simulink model "xeng_8ant"  (Simulink 7.9)
settings: Solver=ode45  StartTime=0.0  StopTime=10.0  RelTol=1e-3
undefined symbols (not defined in the file): casper_library_multipliers, cmult_4bit_em
libraries: xbsIndex_r4 x761, xbsReplacements_r4 x72, casper_library_misc x19, casper_library_correlator x2, casper_library_delays x1
(part 1 of 9)
settings Model: Creator=tfiliba  LastModifiedBy=tfiliba

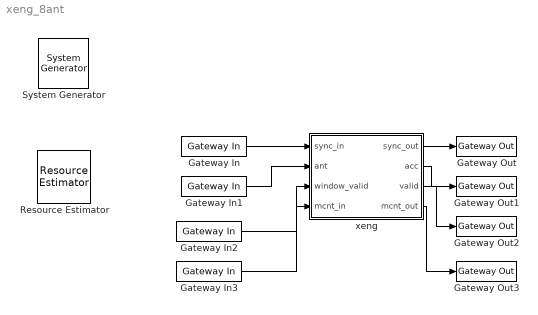
== system xeng_8ant ==
  " System Generator" : xbsIndex_r4/ System Generator  Tag=genX  xilinxfamily=virtex5  part=xc5vsx95t  speed=-1  package=ff1136  synthesis_tool=XST  clock_wrapper=Clock Enables  directory=./netlist  proj_type=Project Navigator  Synth_file=XST Defaults  Impl_file=ISE Defaults  testbench=off  simulink_period=1  sysclk_period=10  dcm_input_clock_period=10  incr_netlist=off  trim_vbits=Everywhere in SubSystem  dbl_ovrd=According to Block Masks  core_generation=According to Block Masks  run_coregen=off  deprecated_control=off  eval_field=0  block_type=sysgen
  Gateway In : xbsIndex_r4/Gateway In  gui_display_data_type=Boolean  arith_type=Boolean  n_bits=16  bin_pt=14  preci_type=Single  exp_width=8  frac_width=24  quantization="Round  (unbiased: +/- Inf)"  overflow=Saturate  period=1  dbl_ovrd=off  timing_constraint=None  locs_specified=off  LOCs={}  UseAsADC=off  ADCChannel='1'  inherit_from_input=off  hdl_port=on  block_type=gatewayin
      settings: xl_area=[0 0 0 0 1 0 0]
  Gateway In1 : xbsIndex_r4/Gateway In  gui_display_data_type=Fixed-point  arith_type="Signed  (2's comp)"  n_bits=32  bin_pt=0  preci_type=Single  exp_width=8  frac_width=24  quantization="Round  (unbiased: +/- Inf)"  overflow=Saturate  period=1  dbl_ovrd=off  timing_constraint=None  locs_specified=off  LOCs={}  UseAsADC=off  ADCChannel='1'  inherit_from_input=off  hdl_port=on  block_type=gatewayin
      settings: xl_area=[0 0 0 0 32 0 0]
  Gateway In2 : xbsIndex_r4/Gateway In  gui_display_data_type=Boolean  arith_type=Boolean  n_bits=4  bin_pt=3  preci_type=Single  exp_width=8  frac_width=24  quantization="Round  (unbiased: +/- Inf)"  overflow=Saturate  period=1  dbl_ovrd=off  timing_constraint=None  locs_specified=off  LOCs={}  UseAsADC=off  ADCChannel='1'  inherit_from_input=off  hdl_port=on  block_type=gatewayin
      settings: xl_area=[0 0 0 0 1 0 0]
  Gateway In3 : xbsIndex_r4/Gateway In  gui_display_data_type=Boolean  arith_type=Boolean  n_bits=4  bin_pt=3  preci_type=Single  exp_width=8  frac_width=24  quantization="Round  (unbiased: +/- Inf)"  overflow=Saturate  period=1  dbl_ovrd=off  timing_constraint=None  locs_specified=off  LOCs={}  UseAsADC=off  ADCChannel='1'  inherit_from_input=off  hdl_port=on  block_type=gatewayin
      settings: xl_area=[0 0 0 0 1 0 0]
  Gateway Out{,1..3} (4 alike) : xbsIndex_r4/Gateway Out  inherit_from_input=off  hdl_port=on  timing_constraint=None  locs_specified=off  LOCs={}  UseAsDAC=off  DACChannel='1'  block_type=gatewayout
      Gateway Out settings: xl_area=[0 0 0 0 1 0 0]
      Gateway Out1 settings: xl_area=[0 0 0 0 16 0 0]
      Gateway Out2 settings: xl_area=[0 0 0 0 1 0 0]
      Gateway Out3 settings: xl_area=[0 0 0 0 1 0 0]
  Resource Estimator : xbsIndex_r4/Resource Estimator  Tag=resEstTag  Slices=4251  FFs=5942  BRAMs=24  LUTs=5653  IOBs=39  EBMs=144  TBUFs=0  xl_use_estimator_area=off  est_options=Estimate  xl_estimator_area="[ 4251  5942    24  5653    39   144     0 ]"  block_type=resource_estimator
      settings: AttributesFormatString=Resource\nEstimator
  xeng : Subsystem  AncestorBlock=casper_library_correlator/xeng  mask(xeng){n_ants=8, n_bits=4, acc_len=128, demux_factor=8, add_latency=1, mult_latency=1, bram_latency=2, use_ded_mult=1, use_bram_delay=1}
      mask prompts: n_ants "Number of antennas"; n_bits "Bit-width of samples in"; acc_len "Accumulation length"; add_latency "Adder latency"; mult_latency "Multiplier latency"; bram_latency "BRAM latency"; use_ded_mult "Implementation: Multiplier type (0=slices 1=embedded 2=bram)"; use_bram_delay "Implementation: Delay type (0=SLR, 1=BRAM)"
      mask help: CASPER X engine with added internal valid data masking functionality, descramble and integral demux. Based on Aaron Parsons' and Lynn Urry's original X engine design.
      mask init:
      | xeng_init(gcb, ...
      |     'n_ants', n_ants, ...
      |     'n_bits', n_bits, ...
      |     'acc_len', acc_len, ...
      |     'demux_factor', demux_factor, ...
      |     'add_latency', add_latency, ...
      |     'mult_latency', mult_latency, ...
      |     'bram_latency', bram_latency, ...
      |     'use_ded_mult', use_ded_mult, ...
      |     'use_bram_delay', use_bram_delay);
      settings: AttributesFormatString=n_ant=8, bits=4, mult=1, bram=1
      mask StyleString: edit,edit,edit,popup(1|2|4|8),edit,edit,edit,edit,edit
  wires:
  Gateway In/1 -> xeng/1(sync_in)
  Gateway In1/1 -> xeng/2(ant)
  Gateway In2/1 -> xeng/3(window_valid)
  Gateway In3/1 -> xeng/4(mcnt_in)
  xeng/1(sync_out) -> Gateway Out/1
  xeng/2(acc) -> Gateway Out1/1
  xeng/3(valid) -> Gateway Out2/1
  xeng/4(mcnt_out) -> Gateway Out3/1

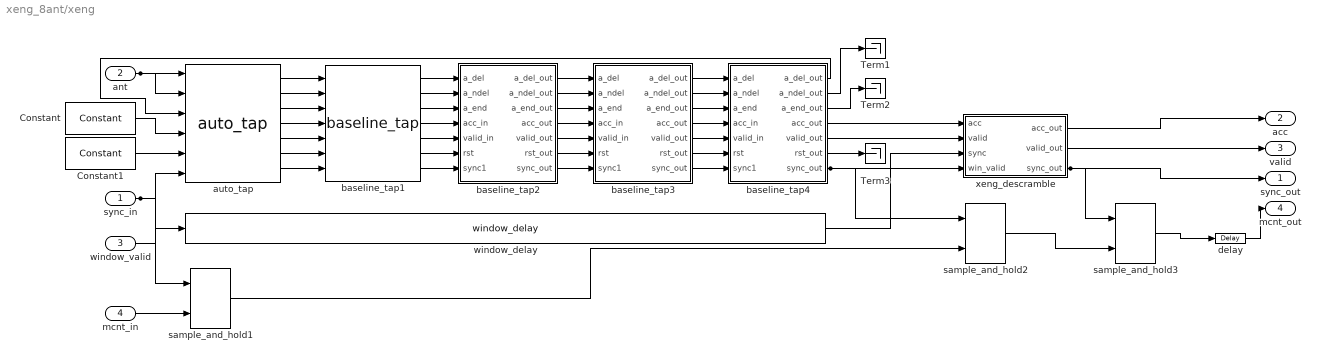
== system xeng_8ant/xeng ==
  sync_in : Inport
  ant : Inport  Port=2
  window_valid : Inport  Port=3
  mcnt_in : Inport  Port=4
  Constant : xbsIndex_r4/Constant  const=0  gui_display_data_type=Fixed-point  arith_type=Unsigned  n_bits=128  bin_pt=14  preci_type=Single  exp_width=8  frac_width=24  explicit_period=off  period=1  equ=P=C  opselect=C  inp2=PCIN>>17  opr=+  inp1=P  carry=CIN  dbl_ovrd=off  block_type=constant
  Constant1 : xbsIndex_r4/Constant  const=0  gui_display_data_type=Fixed-point  arith_type=Boolean  n_bits=1  bin_pt=14  preci_type=Single  exp_width=8  frac_width=24  explicit_period=off  period=1  equ=P=C  opselect=C  inp2=PCIN>>17  opr=+  inp1=P  carry=CIN  dbl_ovrd=off  block_type=constant
  Term1 : Terminator
  Term2 : Terminator
  Term3 : Terminator
  auto_tap : casper_library_correlator/auto_tap  n_ants=8  n_bits=4  acc_len=128  add_latency=1  mult_latency=1  bram_latency=2  use_ded_mult=1  use_bram_delay=1
      link override delay/Counter: use_behavioral_HDL=off  implementation=Fabric  use_rpm=off
      link override dual_pol_cmac/cmac1/cmult*/Resource Estimator: xl_estimator_area=[26 0 0 50 0 4 0]
      link override dual_pol_cmac/cmac2/cmult*/Resource Estimator: xl_estimator_area=[26 0 0 50 0 4 0]
      link override dual_pol_cmac/cmac3/cmult*/Resource Estimator: xl_estimator_area=[26 0 0 50 0 4 0]
      link override dual_pol_cmac/cmac4/cmult*/Resource Estimator: xl_estimator_area=[26 0 0 50 0 4 0]
      settings: AttributesFormatString=mult=1
      link override delay/Counter: xl_area=[8 10 0 13 0 0 0]
      link override delay/Single Port RAM: xl_area=[0 32 8 0 0 0 0]
      link override dual_pol_cmac/cmac1/Counter: xl_area=[6 7 0 9 0 0 0]
      link override dual_pol_cmac/cmac1/Delay: xl_area=[1 1 0 0 0 0 0]
      link override dual_pol_cmac/cmac1/Relational: xl_area=[2 1 0 4 0 0 0]
      link override dual_pol_cmac/cmac1/acc/Accumulator: xl_area=[8 16 0 16 0 0 0]
      link override dual_pol_cmac/cmac1/acc/Convert1: xl_area=[0 0 0 0 0 0 0]
      link override dual_pol_cmac/cmac1/acc/Convert2: xl_area=[0 0 0 0 0 0 0]
      link override dual_pol_cmac/cmac1/acc/Delay: xl_area=[0 0 0 0 0 0 0]
      link override dual_pol_cmac/cmac1/acc/Delay1: xl_area=[0 0 0 0 0 0 0]
      link override dual_pol_cmac/cmac1/acc/Mux2: xl_area=[16 32 0 16 0 0 0]
      link override dual_pol_cmac/cmac1/acc/Mux3: xl_area=[1 2 0 1 0 0 0]
      link override dual_pol_cmac/cmac1/acc1/Accumulator: xl_area=[8 16 0 16 0 0 0]
      link override dual_pol_cmac/cmac1/acc1/Convert1: xl_area=[0 0 0 0 0 0 0]
      link override dual_pol_cmac/cmac1/acc1/Convert2: xl_area=[0 0 0 0 0 0 0]
      link override dual_pol_cmac/cmac1/acc1/Delay: xl_area=[0 0 0 0 0 0 0]
      link override dual_pol_cmac/cmac1/acc1/Delay1: xl_area=[0 0 0 0 0 0 0]
      link override dual_pol_cmac/cmac1/acc1/Mux2: xl_area=[16 32 0 16 0 0 0]
      link override dual_pol_cmac/cmac1/acc1/Mux3: xl_area=[1 2 0 1 0 0 0]
      link override dual_pol_cmac/cmac1/cmult*/ac: xl_area=[4 0 0 8 0 1 0]
      link override dual_pol_cmac/cmac1/cmult*/ad: xl_area=[4 0 0 8 0 1 0]
      link override dual_pol_cmac/cmac1/cmult*/bc: xl_area=[4 0 0 8 0 1 0]
      link override dual_pol_cmac/cmac1/cmult*/bd: xl_area=[4 0 0 8 0 1 0]
      link override dual_pol_cmac/cmac1/cmult*/imag_sum: xl_area=[5 0 0 9 0 0 0]
      link override dual_pol_cmac/cmac1/cmult*/real_sum: xl_area=[5 0 0 9 0 0 0]
      link override dual_pol_cmac/cmac2/Counter: xl_area=[6 7 0 9 0 0 0]
      link override dual_pol_cmac/cmac2/Delay: xl_area=[1 1 0 0 0 0 0]
      link override dual_pol_cmac/cmac2/Relational: xl_area=[2 1 0 4 0 0 0]
      link override dual_pol_cmac/cmac2/acc/Accumulator: xl_area=[8 16 0 16 0 0 0]
      link override dual_pol_cmac/cmac2/acc/Convert1: xl_area=[0 0 0 0 0 0 0]
      link override dual_pol_cmac/cmac2/acc/Convert2: xl_area=[0 0 0 0 0 0 0]
      link override dual_pol_cmac/cmac2/acc/Delay: xl_area=[0 0 0 0 0 0 0]
      link override dual_pol_cmac/cmac2/acc/Delay1: xl_area=[0 0 0 0 0 0 0]
      link override dual_pol_cmac/cmac2/acc/Mux2: xl_area=[16 32 0 16 0 0 0]
      link override dual_pol_cmac/cmac2/acc/Mux3: xl_area=[1 2 0 1 0 0 0]
      link override dual_pol_cmac/cmac2/acc1/Accumulator: xl_area=[8 16 0 16 0 0 0]
      link override dual_pol_cmac/cmac2/acc1/Convert1: xl_area=[0 0 0 0 0 0 0]
      link override dual_pol_cmac/cmac2/acc1/Convert2: xl_area=[0 0 0 0 0 0 0]
      link override dual_pol_cmac/cmac2/acc1/Delay: xl_area=[0 0 0 0 0 0 0]
      link override dual_pol_cmac/cmac2/acc1/Delay1: xl_area=[0 0 0 0 0 0 0]
      link override dual_pol_cmac/cmac2/acc1/Mux2: xl_area=[16 32 0 16 0 0 0]
      link override dual_pol_cmac/cmac2/acc1/Mux3: xl_area=[1 2 0 1 0 0 0]
      link override dual_pol_cmac/cmac2/cmult*/ac: xl_area=[4 0 0 8 0 1 0]
      link override dual_pol_cmac/cmac2/cmult*/ad: xl_area=[4 0 0 8 0 1 0]
      link override dual_pol_cmac/cmac2/cmult*/bc: xl_area=[4 0 0 8 0 1 0]
      link override dual_pol_cmac/cmac2/cmult*/bd: xl_area=[4 0 0 8 0 1 0]
      link override dual_pol_cmac/cmac2/cmult*/imag_sum: xl_area=[5 0 0 9 0 0 0]
      link override dual_pol_cmac/cmac2/cmult*/real_sum: xl_area=[5 0 0 9 0 0 0]
      link override dual_pol_cmac/cmac3/Counter: xl_area=[6 7 0 9 0 0 0]
      link override dual_pol_cmac/cmac3/Delay: xl_area=[1 1 0 0 0 0 0]
      link override dual_pol_cmac/cmac3/Relational: xl_area=[2 1 0 4 0 0 0]
      link override dual_pol_cmac/cmac3/acc/Accumulator: xl_area=[8 16 0 16 0 0 0]
      link override dual_pol_cmac/cmac3/acc/Convert1: xl_area=[0 0 0 0 0 0 0]
      link override dual_pol_cmac/cmac3/acc/Convert2: xl_area=[0 0 0 0 0 0 0]
      link override dual_pol_cmac/cmac3/acc/Delay: xl_area=[0 0 0 0 0 0 0]
      link override dual_pol_cmac/cmac3/acc/Delay1: xl_area=[0 0 0 0 0 0 0]
      link override dual_pol_cmac/cmac3/acc/Mux2: xl_area=[16 32 0 16 0 0 0]
      link override dual_pol_cmac/cmac3/acc/Mux3: xl_area=[1 2 0 1 0 0 0]
      link override dual_pol_cmac/cmac3/acc1/Accumulator: xl_area=[8 16 0 16 0 0 0]
      link override dual_pol_cmac/cmac3/acc1/Convert1: xl_area=[0 0 0 0 0 0 0]
      link override dual_pol_cmac/cmac3/acc1/Convert2: xl_area=[0 0 0 0 0 0 0]
      link override dual_pol_cmac/cmac3/acc1/Delay: xl_area=[0 0 0 0 0 0 0]
      link override dual_pol_cmac/cmac3/acc1/Delay1: xl_area=[0 0 0 0 0 0 0]
      link override dual_pol_cmac/cmac3/acc1/Mux2: xl_area=[16 32 0 16 0 0 0]
      link override dual_pol_cmac/cmac3/acc1/Mux3: xl_area=[1 2 0 1 0 0 0]
      link override dual_pol_cmac/cmac3/cmult*/ac: xl_area=[4 0 0 8 0 1 0]
      link override dual_pol_cmac/cmac3/cmult*/ad: xl_area=[4 0 0 8 0 1 0]
      link override dual_pol_cmac/cmac3/cmult*/bc: xl_area=[4 0 0 8 0 1 0]
      link override dual_pol_cmac/cmac3/cmult*/bd: xl_area=[4 0 0 8 0 1 0]
      link override dual_pol_cmac/cmac3/cmult*/imag_sum: xl_area=[5 0 0 9 0 0 0]
      link override dual_pol_cmac/cmac3/cmult*/real_sum: xl_area=[5 0 0 9 0 0 0]
      link override dual_pol_cmac/cmac4/Counter: xl_area=[6 7 0 9 0 0 0]
      link override dual_pol_cmac/cmac4/Delay: xl_area=[1 1 0 0 0 0 0]
      link override dual_pol_cmac/cmac4/Relational: xl_area=[2 1 0 4 0 0 0]
      link override dual_pol_cmac/cmac4/acc/Accumulator: xl_area=[8 16 0 16 0 0 0]
      link override dual_pol_cmac/cmac4/acc/Convert1: xl_area=[0 0 0 0 0 0 0]
      link override dual_pol_cmac/cmac4/acc/Convert2: xl_area=[0 0 0 0 0 0 0]
      link override dual_pol_cmac/cmac4/acc/Delay: xl_area=[0 0 0 0 0 0 0]
      link override dual_pol_cmac/cmac4/acc/Delay1: xl_area=[0 0 0 0 0 0 0]
      link override dual_pol_cmac/cmac4/acc/Mux2: xl_area=[16 32 0 16 0 0 0]
      link override dual_pol_cmac/cmac4/acc/Mux3: xl_area=[1 2 0 1 0 0 0]
      link override dual_pol_cmac/cmac4/acc1/Accumulator: xl_area=[8 16 0 16 0 0 0]
      link override dual_pol_cmac/cmac4/acc1/Convert1: xl_area=[0 0 0 0 0 0 0]
      link override dual_pol_cmac/cmac4/acc1/Convert2: xl_area=[0 0 0 0 0 0 0]
      link override dual_pol_cmac/cmac4/acc1/Delay: xl_area=[0 0 0 0 0 0 0]
      link override dual_pol_cmac/cmac4/acc1/Delay1: xl_area=[0 0 0 0 0 0 0]
      link override dual_pol_cmac/cmac4/acc1/Mux2: xl_area=[16 32 0 16 0 0 0]
      link override dual_pol_cmac/cmac4/acc1/Mux3: xl_area=[1 2 0 1 0 0 0]
      link override dual_pol_cmac/cmac4/cmult*/ac: xl_area=[4 0 0 8 0 1 0]
      link override dual_pol_cmac/cmac4/cmult*/ad: xl_area=[4 0 0 8 0 1 0]
      link override dual_pol_cmac/cmac4/cmult*/bc: xl_area=[4 0 0 8 0 1 0]
      link override dual_pol_cmac/cmac4/cmult*/bd: xl_area=[4 0 0 8 0 1 0]
      link override dual_pol_cmac/cmac4/cmult*/imag_sum: xl_area=[5 0 0 9 0 0 0]
      link override dual_pol_cmac/cmac4/cmult*/real_sum: xl_area=[5 0 0 9 0 0 0]
      link override sync_delay/Counter: xl_area=[5 8 0 9 0 0 0]
      link override sync_delay/Logical: xl_area=[1 0 0 1 0 0 0]
      link override sync_delay/Mux: xl_area=[1 0 0 1 0 0 0]
      link override sync_delay/Relational: xl_area=[2 0 0 4 0 0 0]
      link override sync_delay/Relational1: xl_area=[2 0 0 4 0 0 0]
  baseline_tap1 : casper_library_correlator/baseline_tap  n_ants=8  ant_sep=1  n_bits=4  acc_len=128  add_latency=1  mult_latency=1  bram_latency=2  use_ded_mult=1  use_bram_delay=1
      link override delay/Counter: use_behavioral_HDL=off  implementation=Fabric  use_rpm=off
      link override dual_pol_cmac/cmac1/cmult*/Resource Estimator: xl_estimator_area=[26 0 0 50 0 4 0]
      link override dual_pol_cmac/cmac2/cmult*/Resource Estimator: xl_estimator_area=[26 0 0 50 0 4 0]
      link override dual_pol_cmac/cmac3/cmult*/Resource Estimator: xl_estimator_area=[26 0 0 50 0 4 0]
      link override dual_pol_cmac/cmac4/cmult*/Resource Estimator: xl_estimator_area=[26 0 0 50 0 4 0]
      settings: AttributesFormatString=ant_sep=1, mult=1, bram=1
      link override Convert: xl_area=[0 0 0 0 0 0 0]
      link override Counter: xl_area=[10 11 0 15 0 0 0]
      link override Delay1: xl_area=[1 1 0 0 0 0 0]
      link override Delay3: xl_area=[16 32 0 0 0 0 0]
      link override Delay7: xl_area=[16 32 0 0 0 0 0]
      link override Delay8: xl_area=[16 32 0 0 0 0 0]
      link override Mux: xl_area=[16 32 0 32 0 0 0]
      link override Relational: xl_area=[6 0 0 11 0 0 0]
      link override delay/Counter: xl_area=[6 7 0 9 0 0 0]
      link override delay/Single Port RAM: xl_area=[0 32 1 0 0 0 0]
      link override dual_pol_cmac/cmac1/Counter: xl_area=[6 7 0 9 0 0 0]
      link override dual_pol_cmac/cmac1/Delay: xl_area=[1 1 0 0 0 0 0]
      link override dual_pol_cmac/cmac1/Relational: xl_area=[2 1 0 4 0 0 0]
      link override dual_pol_cmac/cmac1/acc/Accumulator: xl_area=[8 16 0 16 0 0 0]
      link override dual_pol_cmac/cmac1/acc/Convert1: xl_area=[0 0 0 0 0 0 0]
      link override dual_pol_cmac/cmac1/acc/Convert2: xl_area=[0 0 0 0 0 0 0]
      link override dual_pol_cmac/cmac1/acc/Delay: xl_area=[0 0 0 0 0 0 0]
      link override dual_pol_cmac/cmac1/acc/Delay1: xl_area=[0 0 0 0 0 0 0]
      link override dual_pol_cmac/cmac1/acc/Mux2: xl_area=[16 32 0 16 0 0 0]
      link override dual_pol_cmac/cmac1/acc/Mux3: xl_area=[1 2 0 1 0 0 0]
      link override dual_pol_cmac/cmac1/acc1/Accumulator: xl_area=[8 16 0 16 0 0 0]
      link override dual_pol_cmac/cmac1/acc1/Convert1: xl_area=[0 0 0 0 0 0 0]
      link override dual_pol_cmac/cmac1/acc1/Convert2: xl_area=[0 0 0 0 0 0 0]
      link override dual_pol_cmac/cmac1/acc1/Delay: xl_area=[0 0 0 0 0 0 0]
      link override dual_pol_cmac/cmac1/acc1/Delay1: xl_area=[0 0 0 0 0 0 0]
      link override dual_pol_cmac/cmac1/acc1/Mux2: xl_area=[16 32 0 16 0 0 0]
      link override dual_pol_cmac/cmac1/acc1/Mux3: xl_area=[1 2 0 1 0 0 0]
      link override dual_pol_cmac/cmac1/cmult*/ac: xl_area=[4 0 0 8 0 1 0]
      link override dual_pol_cmac/cmac1/cmult*/ad: xl_area=[4 0 0 8 0 1 0]
      link override dual_pol_cmac/cmac1/cmult*/bc: xl_area=[4 0 0 8 0 1 0]
      link override dual_pol_cmac/cmac1/cmult*/bd: xl_area=[4 0 0 8 0 1 0]
      link override dual_pol_cmac/cmac1/cmult*/imag_sum: xl_area=[5 0 0 9 0 0 0]
      link override dual_pol_cmac/cmac1/cmult*/real_sum: xl_area=[5 0 0 9 0 0 0]
      link override dual_pol_cmac/cmac2/Counter: xl_area=[6 7 0 9 0 0 0]
      link override dual_pol_cmac/cmac2/Delay: xl_area=[1 1 0 0 0 0 0]
      link override dual_pol_cmac/cmac2/Relational: xl_area=[2 1 0 4 0 0 0]
      link override dual_pol_cmac/cmac2/acc/Accumulator: xl_area=[8 16 0 16 0 0 0]
      link override dual_pol_cmac/cmac2/acc/Convert1: xl_area=[0 0 0 0 0 0 0]
      link override dual_pol_cmac/cmac2/acc/Convert2: xl_area=[0 0 0 0 0 0 0]
      link override dual_pol_cmac/cmac2/acc/Delay: xl_area=[0 0 0 0 0 0 0]
      link override dual_pol_cmac/cmac2/acc/Delay1: xl_area=[0 0 0 0 0 0 0]
      link override dual_pol_cmac/cmac2/acc/Mux2: xl_area=[16 32 0 16 0 0 0]
      link override dual_pol_cmac/cmac2/acc/Mux3: xl_area=[1 2 0 1 0 0 0]
      link override dual_pol_cmac/cmac2/acc1/Accumulator: xl_area=[8 16 0 16 0 0 0]
      link override dual_pol_cmac/cmac2/acc1/Convert1: xl_area=[0 0 0 0 0 0 0]
      link override dual_pol_cmac/cmac2/acc1/Convert2: xl_area=[0 0 0 0 0 0 0]
      link override dual_pol_cmac/cmac2/acc1/Delay: xl_area=[0 0 0 0 0 0 0]
      link override dual_pol_cmac/cmac2/acc1/Delay1: xl_area=[0 0 0 0 0 0 0]
      link override dual_pol_cmac/cmac2/acc1/Mux2: xl_area=[16 32 0 16 0 0 0]
      link override dual_pol_cmac/cmac2/acc1/Mux3: xl_area=[1 2 0 1 0 0 0]
      link override dual_pol_cmac/cmac2/cmult*/ac: xl_area=[4 0 0 8 0 1 0]
      link override dual_pol_cmac/cmac2/cmult*/ad: xl_area=[4 0 0 8 0 1 0]
      link override dual_pol_cmac/cmac2/cmult*/bc: xl_area=[4 0 0 8 0 1 0]
      link override dual_pol_cmac/cmac2/cmult*/bd: xl_area=[4 0 0 8 0 1 0]
      link override dual_pol_cmac/cmac2/cmult*/imag_sum: xl_area=[5 0 0 9 0 0 0]
      link override dual_pol_cmac/cmac2/cmult*/real_sum: xl_area=[5 0 0 9 0 0 0]
      link override dual_pol_cmac/cmac3/Counter: xl_area=[6 7 0 9 0 0 0]
      link override dual_pol_cmac/cmac3/Delay: xl_area=[1 1 0 0 0 0 0]
      link override dual_pol_cmac/cmac3/Relational: xl_area=[2 1 0 4 0 0 0]
      link override dual_pol_cmac/cmac3/acc/Accumulator: xl_area=[8 16 0 16 0 0 0]
      link override dual_pol_cmac/cmac3/acc/Convert1: xl_area=[0 0 0 0 0 0 0]
      link override dual_pol_cmac/cmac3/acc/Convert2: xl_area=[0 0 0 0 0 0 0]
      link override dual_pol_cmac/cmac3/acc/Delay: xl_area=[0 0 0 0 0 0 0]
      link override dual_pol_cmac/cmac3/acc/Delay1: xl_area=[0 0 0 0 0 0 0]
      link override dual_pol_cmac/cmac3/acc/Mux2: xl_area=[16 32 0 16 0 0 0]
      link override dual_pol_cmac/cmac3/acc/Mux3: xl_area=[1 2 0 1 0 0 0]
      link override dual_pol_cmac/cmac3/acc1/Accumulator: xl_area=[8 16 0 16 0 0 0]
      link override dual_pol_cmac/cmac3/acc1/Convert1: xl_area=[0 0 0 0 0 0 0]
      link override dual_pol_cmac/cmac3/acc1/Convert2: xl_area=[0 0 0 0 0 0 0]
      link override dual_pol_cmac/cmac3/acc1/Delay: xl_area=[0 0 0 0 0 0 0]
      link override dual_pol_cmac/cmac3/acc1/Delay1: xl_area=[0 0 0 0 0 0 0]
      link override dual_pol_cmac/cmac3/acc1/Mux2: xl_area=[16 32 0 16 0 0 0]
      link override dual_pol_cmac/cmac3/acc1/Mux3: xl_area=[1 2 0 1 0 0 0]
      link override dual_pol_cmac/cmac3/cmult*/ac: xl_area=[4 0 0 8 0 1 0]
      link override dual_pol_cmac/cmac3/cmult*/ad: xl_area=[4 0 0 8 0 1 0]
      link override dual_pol_cmac/cmac3/cmult*/bc: xl_area=[4 0 0 8 0 1 0]
      link override dual_pol_cmac/cmac3/cmult*/bd: xl_area=[4 0 0 8 0 1 0]
      link override dual_pol_cmac/cmac3/cmult*/imag_sum: xl_area=[5 0 0 9 0 0 0]
      link override dual_pol_cmac/cmac3/cmult*/real_sum: xl_area=[5 0 0 9 0 0 0]
      link override dual_pol_cmac/cmac4/Counter: xl_area=[6 7 0 9 0 0 0]
      link override dual_pol_cmac/cmac4/Delay: xl_area=[1 1 0 0 0 0 0]
      link override dual_pol_cmac/cmac4/Relational: xl_area=[2 1 0 4 0 0 0]
      link override dual_pol_cmac/cmac4/acc/Accumulator: xl_area=[8 16 0 16 0 0 0]
      link override dual_pol_cmac/cmac4/acc/Convert1: xl_area=[0 0 0 0 0 0 0]
      link override dual_pol_cmac/cmac4/acc/Convert2: xl_area=[0 0 0 0 0 0 0]
      link override dual_pol_cmac/cmac4/acc/Delay: xl_area=[0 0 0 0 0 0 0]
      link override dual_pol_cmac/cmac4/acc/Delay1: xl_area=[0 0 0 0 0 0 0]
      link override dual_pol_cmac/cmac4/acc/Mux2: xl_area=[16 32 0 16 0 0 0]
      link override dual_pol_cmac/cmac4/acc/Mux3: xl_area=[1 2 0 1 0 0 0]
      link override dual_pol_cmac/cmac4/acc1/Accumulator: xl_area=[8 16 0 16 0 0 0]
      link override dual_pol_cmac/cmac4/acc1/Convert1: xl_area=[0 0 0 0 0 0 0]
      link override dual_pol_cmac/cmac4/acc1/Convert2: xl_area=[0 0 0 0 0 0 0]
      link override dual_pol_cmac/cmac4/acc1/Delay: xl_area=[0 0 0 0 0 0 0]
      link override dual_pol_cmac/cmac4/acc1/Delay1: xl_area=[0 0 0 0 0 0 0]
      link override dual_pol_cmac/cmac4/acc1/Mux2: xl_area=[16 32 0 16 0 0 0]
      link override dual_pol_cmac/cmac4/acc1/Mux3: xl_area=[1 2 0 1 0 0 0]
      link override dual_pol_cmac/cmac4/cmult*/ac: xl_area=[4 0 0 8 0 1 0]
      link override dual_pol_cmac/cmac4/cmult*/ad: xl_area=[4 0 0 8 0 1 0]
      link override dual_pol_cmac/cmac4/cmult*/bc: xl_area=[4 0 0 8 0 1 0]
      link override dual_pol_cmac/cmac4/cmult*/bd: xl_area=[4 0 0 8 0 1 0]
      link override dual_pol_cmac/cmac4/cmult*/imag_sum: xl_area=[5 0 0 9 0 0 0]
      link override dual_pol_cmac/cmac4/cmult*/real_sum: xl_area=[5 0 0 9 0 0 0]
  baseline_tap2 : Subsystem  AncestorBlock=casper_library_correlator/baseline_tap  mask(baseline_tap){n_ants=8, ant_sep=2, n_bits=4, acc_len=128, add_latency=1, mult_latency=1, bram_latency=2, use_ded_mult=1, use_bram_delay=1}
      mask prompts: n_ants "Number of antennas"; ant_sep "Antenna Seperation"; n_bits "number of input bits (per complex component)"; acc_len "accumulation length"; add_latency "Adder latency"; mult_latency "Multiplier latency"; bram_latency "BRAM latency"; use_ded_mult "Multiplier Type (0=slices 1=embedded 2=bram)"; use_bram_delay "Use BRAM delays"
      mask init:
      | fix_pnt_pos = (n_bits-1)*2;
      | bit_growth = ceil(log2(acc_len));
      | ant_bits = ceil(log2(n_ants));
      | n_bits_out = (2*n_bits + 1 + bit_growth);
      | 
      | baseline_tap_init(gcb, ...
      |     'ant_sep', ant_sep, ...
      |     'use_ded_mult', use_ded_mult, ...
      |     'use_bram_delay', use_bram_delay);
      settings: AttributesFormatString=ant_sep=2, mult=1, bram=1
  baseline_tap3 : Subsystem  AncestorBlock=casper_library_correlator/baseline_tap  mask(baseline_tap){n_ants=8, ant_sep=3, n_bits=4, acc_len=128, add_latency=1, mult_latency=1, bram_latency=2, use_ded_mult=1, use_bram_delay=1}
      mask prompts: n_ants "Number of antennas"; ant_sep "Antenna Seperation"; n_bits "number of input bits (per complex component)"; acc_len "accumulation length"; add_latency "Adder latency"; mult_latency "Multiplier latency"; bram_latency "BRAM latency"; use_ded_mult "Multiplier Type (0=slices 1=embedded 2=bram)"; use_bram_delay "Use BRAM delays"
      mask init: same as xeng_8ant/xeng/baseline_tap2
      settings: AttributesFormatString=ant_sep=3, mult=1, bram=1
  baseline_tap4 : Subsystem  AncestorBlock=casper_library_correlator/baseline_tap  mask(baseline_tap){n_ants=8, ant_sep=4, n_bits=4, acc_len=128, add_latency=1, mult_latency=1, bram_latency=2, use_ded_mult=1, use_bram_delay=1}
      mask prompts: n_ants "Number of antennas"; ant_sep "Antenna Seperation"; n_bits "number of input bits (per complex component)"; acc_len "accumulation length"; add_latency "Adder latency"; mult_latency "Multiplier latency"; bram_latency "BRAM latency"; use_ded_mult "Multiplier Type (0=slices 1=embedded 2=bram)"; use_bram_delay "Use BRAM delays"
      mask init: same as xeng_8ant/xeng/baseline_tap2
      settings: AttributesFormatString=ant_sep=4, mult=1, bram=1
  delay : xbsIndex_r4/Delay  rst=off  infoeditControl=Selection of Reset will increase slice count due to use of real FFs and instead of SRLs  en=off  latency=1  dbl_ovrd=off  reg_retiming=on  block_type=delay
  sample_and_hold1 : casper_library_misc/sample_and_hold  period=1024
      link override Counter4: xl_area=[7 11 0 11 0 0 0]
      link override Delay10: xl_area=[1 1 0 0 0 0 0]
      link override Logical: xl_area=[1 0 0 1 0 0 0]
      link override Register: xl_area=[1 1 0 0 0 0 0]
      link override Relational: xl_area=[6 0 0 12 0 0 0]
  sample_and_hold2 : casper_library_misc/sample_and_hold  period=1024
      link override Counter4: xl_area=[7 11 0 11 0 0 0]
      link override Delay10: xl_area=[1 1 0 0 0 0 0]
      link override Logical: xl_area=[1 0 0 1 0 0 0]
      link override Register: xl_area=[1 1 0 0 0 0 0]
      link override Relational: xl_area=[6 0 0 12 0 0 0]
  sample_and_hold3 : casper_library_misc/sample_and_hold  period=1024
      link override Counter4: xl_area=[7 11 0 11 0 0 0]
      link override Delay10: xl_area=[1 1 0 0 0 0 0]
      link override Logical: xl_area=[1 0 0 1 0 0 0]
      link override Register: xl_area=[1 1 0 0 0 0 0]
      link override Relational: xl_area=[6 0 0 12 0 0 0]
  window_delay : casper_library_delays/window_delay  delay=136
      link override Gateway Out2: xl_area=[0 0 0 0 1 0 0]
      link override Gateway Out3: xl_area=[0 0 0 0 1 0 0]
      link override Gateway Out55: xl_area=[0 0 0 0 1 0 0]
      link override Gateway Out56: xl_area=[0 0 0 0 1 0 0]
      link override Register: xl_area=[1 1 0 0 0 0 0]
      link override negedge/Delay: xl_area=[1 1 0 0 0 0 0]
      link override negedge/Inverter: xl_area=[0 0 0 0 0 0 0]
      link override negedge/Logical: xl_area=[1 0 0 1 0 0 0]
      link override posedge3/Delay: xl_area=[1 1 0 0 0 0 0]
      link override posedge3/Inverter: xl_area=[0 0 0 0 0 0 0]
      link override posedge3/Logical: xl_area=[1 0 0 1 0 0 0]
      link override sync_delay/Counter: xl_area=[5 8 0 9 0 0 0]
      link override sync_delay/Logical: xl_area=[1 0 0 1 0 0 0]
      link override sync_delay/Mux: xl_area=[1 0 0 1 0 0 0]
      link override sync_delay/Relational: xl_area=[2 0 0 4 0 0 0]
      link override sync_delay/Relational1: xl_area=[2 0 0 4 0 0 0]
      link override sync_delay1/Counter: xl_area=[5 8 0 9 0 0 0]
      link override sync_delay1/Logical: xl_area=[1 0 0 1 0 0 0]
      link override sync_delay1/Mux: xl_area=[1 0 0 1 0 0 0]
      link override sync_delay1/Relational: xl_area=[2 0 0 4 0 0 0]
      link override sync_delay1/Relational1: xl_area=[2 0 0 4 0 0 0]
  xeng_descramble : Subsystem  AncestorBlock=casper_library_correlator/xeng_descramble  mask(xeng_descramble){num_ants=8, n_bits=4, acc_len=128, demux_factor=8}
      mask prompts: num_ants "Number of Antennas"; n_bits "Input Bitwidth"; acc_len "X engine accumulation length"; demux_factor "Demux Factor"
      mask help:
      | NOT TESTED FOR non-2^N antennas.
      |
      | Descrambles X engine output. Optionally demuxes output.
      mask init:
      | num_taps = floor(num_ants/2) + 1;
      | ant_bits = ceil(log2(num_ants));
      | num_validins = num_ants*num_taps;
      | validin_bits = floor(log2(num_validins))+1;
      | demux_bits = floor(log2(demux_factor))+1;
      | acc_len_bits = floor(log2(acc_len))+1;
      | num_ants_bits = floor(log2(num_ants))+1;
      | taps_bits = floor(log2(num_taps))+1;
      | pivot_pnt = num_ants/2*(num_taps) + num_taps*num_ants/4;
      | num_elements = nchoosek(num_ants, 2) + num_ants;
      | elements_bits = floor(log2(num_elements)) + 1;
      | n_bits_xeng_out = (2*n_bits + acc_len_bits);
      | n_bits_in = 2^(ceil(log2(n_bits_xeng_out)))*8;
      | 
      | ship_el_del = floor(acc_len*num_ants/num_validins/demux_factor) - 1;
      | 
      | if (ship_el_del < 0)
      |     errordlg('Insufficient output space for this configuration. Try a lower demux setting. Else you need fewer antennas or longer xeng acc time.');
      |     ship_el_del=0;
      | end
      | 
      | if (ship_el_del == 0)
      |     ship_el_cnt = demux_factor*num_elements-1;
      |     %in this case we're outputting multiple words back-to-back.
      | else
      |     ship_el_cnt = demux_factor*num_elements;
      |     %in this case we're outputting one word at a time.
      | end
      | 
      | ship_el_del_bits = ceil(log2(ship_el_del + 1));
      | 
      | if (ship_el_del_bits == 0)
      |     ship_el_del_bits =1;
      | end
      | 
      | fmtstr = sprintf('num_ants=%d',num_ants);
      | set_param(gcb, 'AttributesFormatString', fmtstr);
      settings: AttributesFormatString=num_ants=8
  sync_out : Outport
  acc : Outport  Port=2
  valid : Outport  Port=3
  mcnt_out : Outport  Port=4
  wires:
  xeng_descramble/1(acc_out) -> acc/1
  xeng_descramble/2(valid_out) -> valid/1
  xeng_descramble/3(sync_out) -> sync_out/1, sample_and_hold3/1
  baseline_tap4/4(acc_out) -> xeng_descramble/1(acc)
  baseline_tap4/5(valid_out) -> xeng_descramble/2(valid)
  baseline_tap4/7(sync_out) -> xeng_descramble/3(sync), sample_and_hold2/1
  window_delay/1 -> xeng_descramble/4(win_valid)
  ant/1 -> auto_tap/1, auto_tap/2
  Constant/1 -> auto_tap/4
  Constant1/1 -> auto_tap/5
  sync_in/1 -> auto_tap/6, sample_and_hold1/1
  window_valid/1 -> window_delay/1
  mcnt_in/1 -> sample_and_hold1/2
  sample_and_hold1/1 -> sample_and_hold2/2
  sample_and_hold2/1 -> sample_and_hold3/2
  sample_and_hold3/1 -> delay/1
  delay/1 -> mcnt_out/1
  auto_tap/1 -> baseline_tap1/1
  auto_tap/2 -> baseline_tap1/2
  auto_tap/3 -> baseline_tap1/3
  auto_tap/4 -> baseline_tap1/4
  auto_tap/5 -> baseline_tap1/5
  auto_tap/6 -> baseline_tap1/6
  auto_tap/7 -> baseline_tap1/7
  baseline_tap1/1 -> baseline_tap2/1(a_del)
  baseline_tap1/2 -> baseline_tap2/2(a_ndel)
  baseline_tap1/3 -> baseline_tap2/3(a_end)
  baseline_tap1/4 -> baseline_tap2/4(acc_in)
  baseline_tap1/5 -> baseline_tap2/5(valid_in)
  baseline_tap1/6 -> baseline_tap2/6(rst)
  baseline_tap1/7 -> baseline_tap2/7(sync1)
  baseline_tap2/1(a_del_out) -> baseline_tap3/1(a_del)
  baseline_tap2/2(a_ndel_out) -> baseline_tap3/2(a_ndel)
  baseline_tap2/3(a_end_out) -> baseline_tap3/3(a_end)
  baseline_tap2/4(acc_out) -> baseline_tap3/4(acc_in)
  baseline_tap2/5(valid_out) -> baseline_tap3/5(valid_in)
  baseline_tap2/6(rst_out) -> baseline_tap3/6(rst)
  baseline_tap2/7(sync_out) -> baseline_tap3/7(sync1)
  baseline_tap3/1(a_del_out) -> baseline_tap4/1(a_del)
  baseline_tap3/2(a_ndel_out) -> baseline_tap4/2(a_ndel)
  baseline_tap3/3(a_end_out) -> baseline_tap4/3(a_end)
  baseline_tap3/4(acc_out) -> baseline_tap4/4(acc_in)
  baseline_tap3/5(valid_out) -> baseline_tap4/5(valid_in)
  baseline_tap3/6(rst_out) -> baseline_tap4/6(rst)
  baseline_tap3/7(sync_out) -> baseline_tap4/7(sync1)
  baseline_tap4/1(a_del_out) -> auto_tap/3
  baseline_tap4/2(a_ndel_out) -> Term1/1
  baseline_tap4/3(a_end_out) -> Term2/1
  baseline_tap4/6(rst_out) -> Term3/1

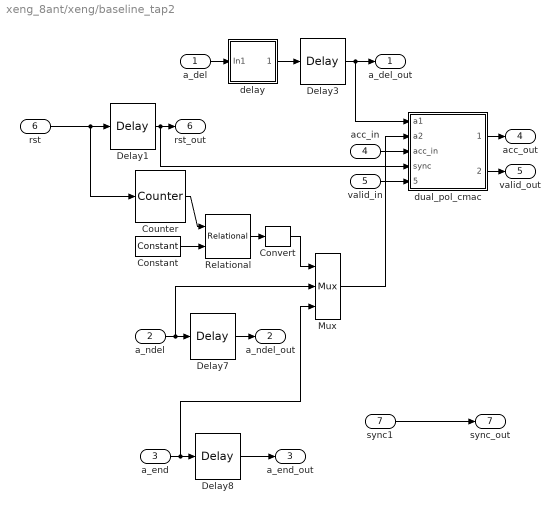
== system xeng_8ant/xeng/baseline_tap2 ==
  a_del : Inport
  a_ndel : Inport  Port=2
  a_end : Inport  Port=3
  acc_in : Inport  Port=4
  valid_in : Inport  Port=5
  rst : Inport  Port=6
  sync1 : Inport  Port=7
  Constant : xbsIndex_r4/Constant  const=ant_sep * acc_len  gui_display_data_type=Fixed-point  arith_type=Unsigned  n_bits=ant_bits + bit_growth  bin_pt=0  preci_type=Single  exp_width=8  frac_width=24  explicit_period=off  period=1  equ=P=C  opselect=C  inp2=PCIN>>17  opr=+  inp1=P  carry=CIN  dbl_ovrd=off  block_type=constant
      settings: block_version=9.1.01
  Convert : xbsIndex_r4/Convert  gui_display_data_type=Fixed-point  arith_type=Unsigned  n_bits=1  bin_pt=0  float_type=Single  exp_bits=8  fraction_bits=24  quantization=Truncate  overflow=Wrap  en=off  latency=0  dbl_ovrd=off  pipeline=off  block_type=convert
      settings: xl_area=[0 0 0 0 0 0 0]
  Counter : xbsIndex_r4/Counter  cnt_type=Count Limited  cnt_to=n_ants * acc_len - 1  operation=Up  start_count=0  cnt_by_val=1  arith_type=Unsigned  n_bits=ant_bits + bit_growth  bin_pt=0  load_pin=off  rst=on  en=off  explicit_period=off  period=1  dbl_ovrd=off  use_behavioral_HDL=off  implementation=Fabric  use_rpm=on  block_type=counter
      settings: xl_area=[10 11 0 15 0 0 0]  block_version=9.1.01
  Delay{1,3,7..8} (4 alike) : xbsIndex_r4/Delay  rst=off  infoeditControl=Selection of Reset will increase slice count due to use of real FFs and instead of SRLs  en=off  latency=1  dbl_ovrd=off  reg_retiming=on  block_type=delay
      Delay1 settings: xl_area=[1 1 0 0 0 0 0]  block_version=9.1.01
      Delay3 settings: xl_area=[16 32 0 0 0 0 0]  block_version=9.1.01
      Delay7 settings: xl_area=[16 32 0 0 0 0 0]  block_version=9.1.01
      Delay8 settings: xl_area=[16 32 0 0 0 0 0]  block_version=9.1.01
  Mux : xbsIndex_r4/Mux  inputs=2  en=off  latency=1  precision=Full  arith_type="Signed  (2's comp)"  n_bits=8  bin_pt=2  quantization=Truncate  overflow=Wrap  dbl_ovrd=off  block_type=mux
      settings: xl_area=[16 32 0 32 0 0 0]  block_version=9.1.01
  Relational : xbsIndex_r4/Relational  mode=a<b  en=off  latency=0  dbl_ovrd=off  block_type=relational
      settings: xl_area=[6 0 0 11 0 0 0]  block_version=9.1.01
  delay : Subsystem  AncestorBlock=casper_library_delays/delay_bram  mask(delay_bram){DelayLen=acc_len, bram_latency=bram_latency, use_dsp48=off}
      mask prompts: DelayLen "Delay By:"; bram_latency "BRAM Latency"; use_dsp48 "Use DSP48"
      mask help: A delay block that uses BRAM for its storage.
      mask init:
      | if (DelayLen <= bram_latency)
      | 	error('delay value must be greater than BRAM Latency');
      | end
      | BitWidth = max(ceil(log2(DelayLen)), 2);
      | if strcmp(use_dsp48,'on'),
      |     set_param([gcb,'/Counter'], 'use_behavioral_HDL', 'off', ...
      |         'use_rpm', 'on', 'implementation', 'DSP48');
      | else, %default counter settings
      |         set_param([gcb,'/Counter'], 'use_behavioral_HDL', 'off', ...
      |         'use_rpm', 'off', 'implementation', 'Fabric');
      | end
      mask Help: eval('xlWeb(''http://casper.berkeley.edu/wiki/Delay_bram'')')
  dual_pol_cmac : Subsystem
  a_del_out : Outport
  a_ndel_out : Outport  Port=2
  a_end_out : Outport  Port=3
  acc_out : Outport  Port=4
  valid_out : Outport  Port=5
  rst_out : Outport  Port=6
  sync_out : Outport  Port=7
  wires:
  delay/1(Out1) -> Delay3/1
  Mux/1 -> dual_pol_cmac/2(a2)
  Counter/1 -> Relational/1
  Constant/1 -> Relational/2
  Relational/1 -> Convert/1
  Convert/1 -> Mux/1
  rst/1 -> Delay1/1, Counter/1
  a_del/1 -> delay/1(In1)
  dual_pol_cmac/1(acc_out) -> acc_out/1
  acc_in/1 -> dual_pol_cmac/3(acc_in)
  dual_pol_cmac/2(valid_out) -> valid_out/1
  valid_in/1 -> dual_pol_cmac/5(valid_in)
  a_ndel/1 -> Mux/2, Delay7/1
  a_end/1 -> Mux/3, Delay8/1
  Delay3/1 -> dual_pol_cmac/1(a1), a_del_out/1
  Delay7/1 -> a_ndel_out/1
  Delay8/1 -> a_end_out/1
  Delay1/1 -> dual_pol_cmac/4(sync), rst_out/1
  sync1/1 -> sync_out/1

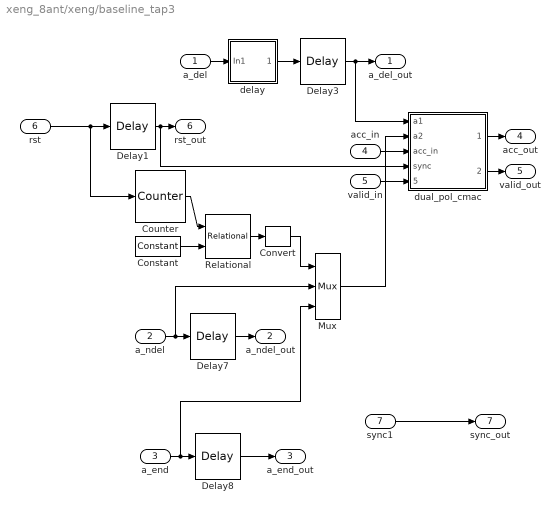
== system xeng_8ant/xeng/baseline_tap3 ==
  a_del : Inport
  a_ndel : Inport  Port=2
  a_end : Inport  Port=3
  acc_in : Inport  Port=4
  valid_in : Inport  Port=5
  rst : Inport  Port=6
  sync1 : Inport  Port=7
  Constant : xbsIndex_r4/Constant  const=ant_sep * acc_len  gui_display_data_type=Fixed-point  arith_type=Unsigned  n_bits=ant_bits + bit_growth  bin_pt=0  preci_type=Single  exp_width=8  frac_width=24  explicit_period=off  period=1  equ=P=C  opselect=C  inp2=PCIN>>17  opr=+  inp1=P  carry=CIN  dbl_ovrd=off  block_type=constant
      settings: block_version=9.1.01
  Convert : xbsIndex_r4/Convert  gui_display_data_type=Fixed-point  arith_type=Unsigned  n_bits=1  bin_pt=0  float_type=Single  exp_bits=8  fraction_bits=24  quantization=Truncate  overflow=Wrap  en=off  latency=0  dbl_ovrd=off  pipeline=off  block_type=convert
      settings: xl_area=[0 0 0 0 0 0 0]
  Counter : xbsIndex_r4/Counter  cnt_type=Count Limited  cnt_to=n_ants * acc_len - 1  operation=Up  start_count=0  cnt_by_val=1  arith_type=Unsigned  n_bits=ant_bits + bit_growth  bin_pt=0  load_pin=off  rst=on  en=off  explicit_period=off  period=1  dbl_ovrd=off  use_behavioral_HDL=off  implementation=Fabric  use_rpm=on  block_type=counter
      settings: xl_area=[10 11 0 15 0 0 0]  block_version=9.1.01
  Delay{1,3,7..8} (4 alike) : xbsIndex_r4/Delay  rst=off  infoeditControl=Selection of Reset will increase slice count due to use of real FFs and instead of SRLs  en=off  latency=1  dbl_ovrd=off  reg_retiming=on  block_type=delay
      Delay1 settings: xl_area=[1 1 0 0 0 0 0]  block_version=9.1.01
      Delay3 settings: xl_area=[16 32 0 0 0 0 0]  block_version=9.1.01
      Delay7 settings: xl_area=[16 32 0 0 0 0 0]  block_version=9.1.01
      Delay8 settings: xl_area=[16 32 0 0 0 0 0]  block_version=9.1.01
  Mux : xbsIndex_r4/Mux  inputs=2  en=off  latency=1  precision=Full  arith_type="Signed  (2's comp)"  n_bits=8  bin_pt=2  quantization=Truncate  overflow=Wrap  dbl_ovrd=off  block_type=mux
      settings: xl_area=[16 32 0 32 0 0 0]  block_version=9.1.01
  Relational : xbsIndex_r4/Relational  mode=a<b  en=off  latency=0  dbl_ovrd=off  block_type=relational
      settings: xl_area=[6 0 0 11 0 0 0]  block_version=9.1.01
  delay : Subsystem  AncestorBlock=casper_library_delays/delay_bram  mask(delay_bram){DelayLen=acc_len, bram_latency=bram_latency, use_dsp48=off}
      mask prompts: DelayLen "Delay By:"; bram_latency "BRAM Latency"; use_dsp48 "Use DSP48"
      mask help: A delay block that uses BRAM for its storage.
      mask init: same as xeng_8ant/xeng/baseline_tap2/delay
      mask Help: eval('xlWeb(''http://casper.berkeley.edu/wiki/Delay_bram'')')
  dual_pol_cmac : Subsystem
  a_del_out : Outport
  a_ndel_out : Outport  Port=2
  a_end_out : Outport  Port=3
  acc_out : Outport  Port=4
  valid_out : Outport  Port=5
  rst_out : Outport  Port=6
  sync_out : Outport  Port=7
  wires:
  delay/1(Out1) -> Delay3/1
  Mux/1 -> dual_pol_cmac/2(a2)
  Counter/1 -> Relational/1
  Constant/1 -> Relational/2
  Relational/1 -> Convert/1
  Convert/1 -> Mux/1
  rst/1 -> Delay1/1, Counter/1
  a_del/1 -> delay/1(In1)
  dual_pol_cmac/1(acc_out) -> acc_out/1
  acc_in/1 -> dual_pol_cmac/3(acc_in)
  dual_pol_cmac/2(valid_out) -> valid_out/1
  valid_in/1 -> dual_pol_cmac/5(valid_in)
  a_ndel/1 -> Mux/2, Delay7/1
  a_end/1 -> Mux/3, Delay8/1
  Delay3/1 -> dual_pol_cmac/1(a1), a_del_out/1
  Delay7/1 -> a_ndel_out/1
  Delay8/1 -> a_end_out/1
  Delay1/1 -> dual_pol_cmac/4(sync), rst_out/1
  sync1/1 -> sync_out/1

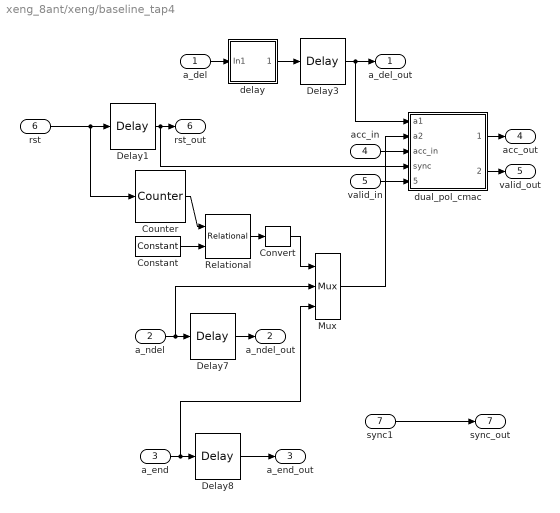
== system xeng_8ant/xeng/baseline_tap4 ==
  a_del : Inport
  a_ndel : Inport  Port=2
  a_end : Inport  Port=3
  acc_in : Inport  Port=4
  valid_in : Inport  Port=5
  rst : Inport  Port=6
  sync1 : Inport  Port=7
  Constant : xbsIndex_r4/Constant  const=ant_sep * acc_len  gui_display_data_type=Fixed-point  arith_type=Unsigned  n_bits=ant_bits + bit_growth  bin_pt=0  preci_type=Single  exp_width=8  frac_width=24  explicit_period=off  period=1  equ=P=C  opselect=C  inp2=PCIN>>17  opr=+  inp1=P  carry=CIN  dbl_ovrd=off  block_type=constant
      settings: block_version=9.1.01
  Convert : xbsIndex_r4/Convert  gui_display_data_type=Fixed-point  arith_type=Unsigned  n_bits=1  bin_pt=0  float_type=Single  exp_bits=8  fraction_bits=24  quantization=Truncate  overflow=Wrap  en=off  latency=0  dbl_ovrd=off  pipeline=off  block_type=convert
      settings: xl_area=[0 0 0 0 0 0 0]
  Counter : xbsIndex_r4/Counter  cnt_type=Count Limited  cnt_to=n_ants * acc_len - 1  operation=Up  start_count=0  cnt_by_val=1  arith_type=Unsigned  n_bits=ant_bits + bit_growth  bin_pt=0  load_pin=off  rst=on  en=off  explicit_period=off  period=1  dbl_ovrd=off  use_behavioral_HDL=off  implementation=Fabric  use_rpm=on  block_type=counter
      settings: xl_area=[10 11 0 15 0 0 0]  block_version=9.1.01
  Delay{1,3,7..8} (4 alike) : xbsIndex_r4/Delay  rst=off  infoeditControl=Selection of Reset will increase slice count due to use of real FFs and instead of SRLs  en=off  latency=1  dbl_ovrd=off  reg_retiming=on  block_type=delay
      Delay1 settings: xl_area=[1 1 0 0 0 0 0]  block_version=9.1.01
      Delay3 settings: xl_area=[16 32 0 0 0 0 0]  block_version=9.1.01
      Delay7 settings: xl_area=[16 32 0 0 0 0 0]  block_version=9.1.01
      Delay8 settings: xl_area=[16 32 0 0 0 0 0]  block_version=9.1.01
  Mux : xbsIndex_r4/Mux  inputs=2  en=off  latency=1  precision=Full  arith_type="Signed  (2's comp)"  n_bits=8  bin_pt=2  quantization=Truncate  overflow=Wrap  dbl_ovrd=off  block_type=mux
      settings: xl_area=[16 32 0 32 0 0 0]  block_version=9.1.01
  Relational : xbsIndex_r4/Relational  mode=a<b  en=off  latency=0  dbl_ovrd=off  block_type=relational
      settings: xl_area=[6 0 0 11 0 0 0]  block_version=9.1.01
  delay : Subsystem  AncestorBlock=casper_library_delays/delay_bram  mask(delay_bram){DelayLen=acc_len, bram_latency=bram_latency, use_dsp48=off}
      mask prompts: DelayLen "Delay By:"; bram_latency "BRAM Latency"; use_dsp48 "Use DSP48"
      mask help: A delay block that uses BRAM for its storage.
      mask init: same as xeng_8ant/xeng/baseline_tap2/delay
      mask Help: eval('xlWeb(''http://casper.berkeley.edu/wiki/Delay_bram'')')
  dual_pol_cmac : Subsystem
  a_del_out : Outport
  a_ndel_out : Outport  Port=2
  a_end_out : Outport  Port=3
  acc_out : Outport  Port=4
  valid_out : Outport  Port=5
  rst_out : Outport  Port=6
  sync_out : Outport  Port=7
  wires:
  delay/1(Out1) -> Delay3/1
  Mux/1 -> dual_pol_cmac/2(a2)
  Counter/1 -> Relational/1
  Constant/1 -> Relational/2
  Relational/1 -> Convert/1
  Convert/1 -> Mux/1
  rst/1 -> Delay1/1, Counter/1
  a_del/1 -> delay/1(In1)
  dual_pol_cmac/1(acc_out) -> acc_out/1
  acc_in/1 -> dual_pol_cmac/3(acc_in)
  dual_pol_cmac/2(valid_out) -> valid_out/1
  valid_in/1 -> dual_pol_cmac/5(valid_in)
  a_ndel/1 -> Mux/2, Delay7/1
  a_end/1 -> Mux/3, Delay8/1
  Delay3/1 -> dual_pol_cmac/1(a1), a_del_out/1
  Delay7/1 -> a_ndel_out/1
  Delay8/1 -> a_end_out/1
  Delay1/1 -> dual_pol_cmac/4(sync), rst_out/1
  sync1/1 -> sync_out/1
